simulink model "punto_cc_simulink_200901"  (R2019a)
settings: Solver=VariableStepAuto  StartTime=0.0  StopTime=600*2*pi  RelTol=1e-3
libraries: cstblocks x2
settings Model: Creator=Marco Greco  LastModifiedBy=Marco Greco

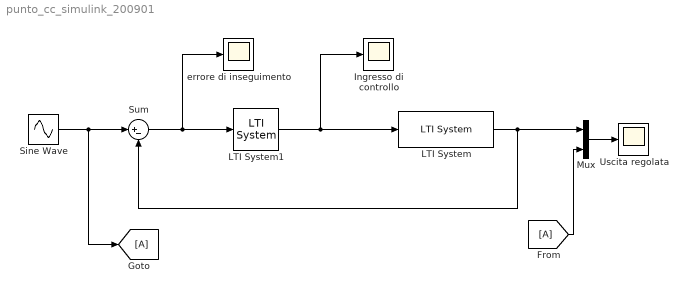
== system punto_cc_simulink_200901 ==
  Ingresso di controllo : Scope
  LTI System : cstblocks/LTI System  sys=G  IC=[]
  LTI System1 : cstblocks/LTI System  sys=C  IC=[]
  Mux : Mux  Inputs=2
  Sine Wave : Sin  Frequency=1/12  SampleTime=0
  Sum : Sum  Inputs=|+-
  Uscita regolata : Scope
  "errore di inseguimento " : Scope
  wires:
  Sine Wave/1 -> [A], Sum/1
  Sum/1 -> LTI System1/1, "errore di inseguimento "/1
  LTI System1/1 -> LTI System/1, Ingresso di controllo/1
  LTI System/1 -> Sum/2, Mux/1
  Mux/1 -> Uscita regolata/1
  [A] -> Mux/2
